simulink model "mod7a"  (Simulink 7.8)
settings: Solver=ode45  StartTime=0.0  StopTime=4  RelTol=1e-3
settings Model: Creator=2017051165  LastModifiedBy=2017051165
settings DebuggingCC: FcnCallInpInsideContextMsg=Use local settings  StrictBusMsg=Warning

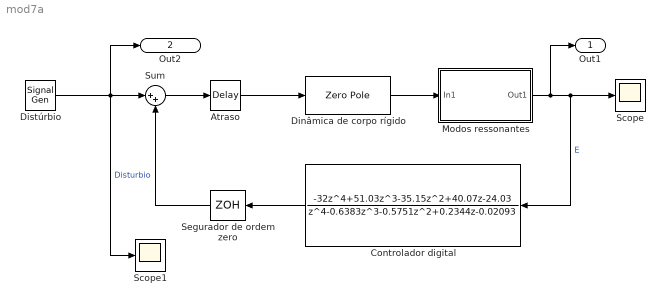
== system mod7a ==
  Atraso : TransportDelay
  Controlador digital : DiscreteTransferFcn  Numerator=[-32 51.03 -35.15 40.07 -24.03]  Denominator=[1 -0.6383 -0.5751 0.2344 -0.02093]  SampleTime=70e-6
  Dinâmica de corpo rígido : ZeroPole  Zeros=[0]  Poles=[0 -12.5]  Gain=[1e6]
  Distúrbio : SignalGenerator  WaveForm=square  Amplitude=20  Frequency=0.325
  Modos ressonantes : Subsystem
  Scope : Scope
      settings: YMin=-1000  YMax=1000  Decimation=200
  Scope1 : Scope
      settings: YMin=-1000  YMax=1000  Decimation=200
  Segurador de ordem zero : ZeroOrderHold  SampleTime=-1
  Sum : Sum  Inputs=|++
  Out1 : Outport
  Out2 : Outport  Port=2
  wires:
  Segurador de ordem zero/1 -> Sum/2
  Distúrbio/1 -> Sum/1, Out2/1, Scope1/1  "Disturbio"
  Sum/1 -> Atraso/1
  Atraso/1 -> Dinâmica de corpo rígido/1
  Controlador digital/1 -> Segurador de ordem zero/1
  Dinâmica de corpo rígido/1 -> Modos ressonantes/1(In1)
  Modos ressonantes/1(Out1) -> Scope/1, Controlador digital/1, Out1/1  "E"

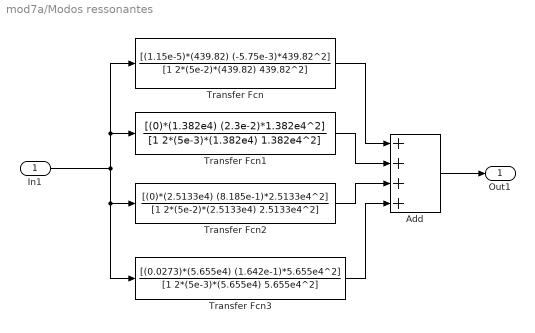
== system mod7a/Modos ressonantes ==
  In1 : Inport
  Add : Sum  Inputs=++++
  Transfer Fcn : TransferFcn  Numerator=[(1.15e-5)*(439.82) (-5.75e-3)*439.82^2]  Denominator=[1 2*(5e-2)*(439.82) 439.82^2]
  Transfer Fcn1 : TransferFcn  Numerator=[(0)*(1.382e4) (2.3e-2)*1.382e4^2]  Denominator=[1 2*(5e-3)*(1.382e4) 1.382e4^2]
  Transfer Fcn2 : TransferFcn  Numerator=[(0)*(2.5133e4) (8.185e-1)*2.5133e4^2]  Denominator=[1 2*(5e-2)*(2.5133e4) 2.5133e4^2]
  Transfer Fcn3 : TransferFcn  Numerator=[(0.0273)*(5.655e4) (1.642e-1)*5.655e4^2]  Denominator=[1 2*(5e-3)*(5.655e4) 5.655e4^2]
  Out1 : Outport
  wires:
  Transfer Fcn3/1 -> Add/4
  Transfer Fcn2/1 -> Add/3
  Transfer Fcn1/1 -> Add/2
  Transfer Fcn/1 -> Add/1
  In1/1 -> Transfer Fcn/1, Transfer Fcn1/1, Transfer Fcn2/1, Transfer Fcn3/1
  Add/1 -> Out1/1
